simulink model "TerrainSimRunner"  (R2021a)
settings: Solver=VariableStepAuto  StartTime=0.0  StopTime=10.6  RelTol=1e-3
values from neighbouring files (symbols this model uses):
  init_parameters = struct    [TerrainGenerator.m]    (also in WorkspaceLoader.m = load('init_parameters'))
undefined symbols (not defined in the file or in its folder): Xref
libraries: vrlib x3
settings Model: Creator=16109  LastModifiedBy=16109

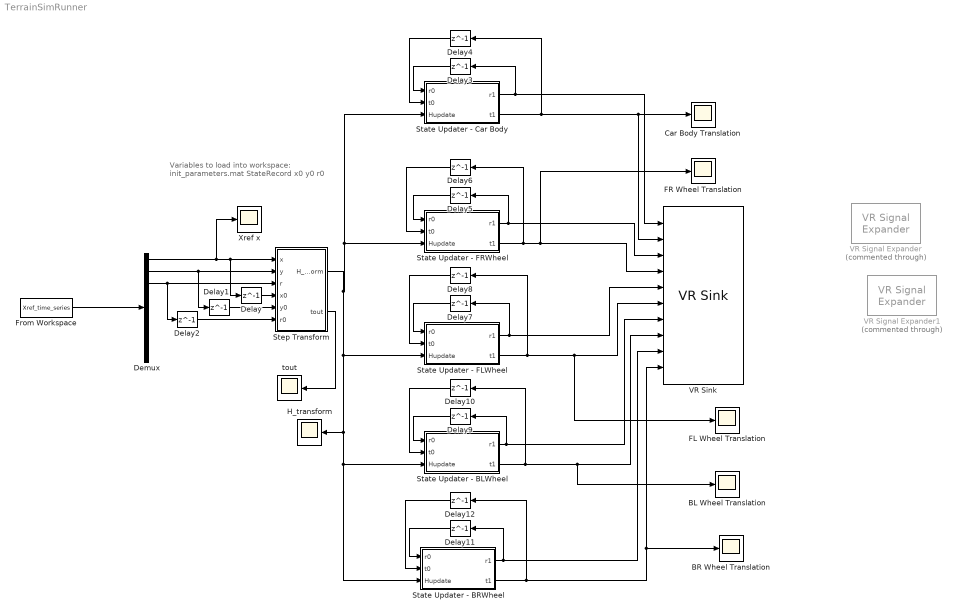
== system TerrainSimRunner ==
  note: Variables to load into workspace:
      | init_parameters.mat
      | StateRecord
      | x0
      | y0
      | r0
  BL Wheel Translation : Scope
  BR Wheel Translation : Scope
  Car Body Translation : Scope
  Delay : Delay  DelayLength=1  InitialCondition=Xref(1,1)
  Delay1 : Delay  DelayLength=1  InitialCondition=Xref(2,1)
  Delay10 : Delay  DelayLength=1  InitialCondition=init_parameters.BLWheelTranslation
  Delay11 : Delay  DelayLength=1  InitialCondition=init_parameters.BRWheelRotation
  Delay12 : Delay  DelayLength=1  InitialCondition=init_parameters.BLWheelTranslation
  Delay2 : Delay  DelayLength=1  InitialCondition=Xref(3,1)
  Delay3 : Delay  DelayLength=1  InitialCondition=init_parameters.BodyRotation
  Delay4 : Delay  DelayLength=1  InitialCondition=init_parameters.BodyTranslation
  Delay5 : Delay  DelayLength=1  InitialCondition=init_parameters.FRWheelRotation
  Delay6 : Delay  DelayLength=1  InitialCondition=init_parameters.FRWheelTranslation
  Delay7 : Delay  DelayLength=1  InitialCondition=init_parameters.FLWheelRotation
  Delay8 : Delay  DelayLength=1  InitialCondition=init_parameters.FLWheelTranslation
  Delay9 : Delay  DelayLength=1  InitialCondition=init_parameters.BLWheelRotation
  Demux : Demux  Outputs=9
  FL Wheel Translation : Scope
  FR Wheel Translation : Scope
  From Workspace : FromWorkspace  VariableName=Xref_time_series
  H_transform : Scope
  State Updater - BLWheel : MATLAB Function  TreatAsAtomicUnit=on
  State Updater - BRWheel : MATLAB Function  TreatAsAtomicUnit=on
  State Updater - Car Body : MATLAB Function  TreatAsAtomicUnit=on
  State Updater - FLWheel : MATLAB Function  TreatAsAtomicUnit=on
  State Updater - FRWheel : MATLAB Function  TreatAsAtomicUnit=on
  Step Transform : MATLAB Function  TreatAsAtomicUnit=on
  VR Signal Expander : vrlib/VR Signal Expander  Commented=through  outwidth=4  outidx=[2 4]
  VR Signal Expander1 : vrlib/VR Signal Expander  Commented=through  outwidth=3  outidx=[1]
  VR Sink : vrlib/VR Sink  InstantiateOnLoad=on  SampleTime=0.1  ViewEnable=on  RemoteChange=off  RemoteView=off  FieldsWritten=CarBody.rotation.4.1.1.double#CarBody.translation.3.1.1.double#FRWheel.rotation.4.1.1.double#FRWheel.translation.3.1.1.double#FLWheel.rotation.4.1.1.double#FLWheel.translation.3.1.1.double#BLWheel.rotation.4.1.1.double#BLWheel.translation.3.1.1.double#BRWheel.rotation.4.1.1.double#BRWheel.translation.3.1.1.double  WorldFileName=TerrainSimulation.x3d  AutoView=off  VideoDimensions=[]  AllowVariableSize=off  FigureProperties="{'Position', 'Name', 'Viewpoint', 'CameraBound', 'CameraDirection', 'CameraPosition', 'CameraUpVector', 'ZoomFactor', 'Antialiasing', 'Headlight', 'Lighting', 'NavPanel', 'Sound', 'StatusBar', 'Stereo3D', 'Stereo3DCameraOffset', 'Stereo3DHIT', 'ToolBar', 'Textures', 'Transparency', 'Triad', 'Wireframe', 'NavZones', 'NavMode', 'NavSpeed', 'CaptureFileFormat', 'CaptureFileName', 'Record2DCompressMethod', 'Record2DCompressQuality', 'Record2D', 'Record2DFileName', 'Record2DFPS'; [5.0000000000000000e+00   9.2000000000000000e+01   5.7600000000000000e+02   3.5000000000000000e+02], '', 'Terrain_Viewpoint_1', 'on', [-6.3529519425843139e-01   3.7869028019551818e-02  -7.7134036123425920e-01], [8.6325161926899163e+00  -2.3623592187623753e+01  -3.9838539482567555e+01], [-3.3509979340254042e-02   9.9650453597280886e-01   7.6523140750056506e-02], [1.0000000000000000e+00], 'off', 'on', 'on', 'halfbar', 'on', 'on', 'off', [1.0000000149011612e-01], [0.0000000000000000e+00], 'on', 'on', 'on', 'none', 'off', 'off', 'examine', 'normal', 'tif', '%f_anim_%n.tif', 'auto', [7.5000000000000000e+01], 'off', '%f_anim_%n.avi', 'auto'}"
  Xref x : Scope
  tout : Scope
  wires:
  From Workspace/1 -> Demux/1
  Demux/1 -> Xref x/1, Delay/1, Step Transform/1(x)
  Demux/2 -> Delay1/1, Step Transform/2(y)
  Demux/3 -> Delay2/1, Step Transform/3(r)
  Delay/1 -> Step Transform/4(x0)
  Delay1/1 -> Step Transform/5(y0)
  Delay2/1 -> Step Transform/6(r0)
  Step Transform/1(H_transform) -> H_transform/1, State Updater - BRWheel/3(Hupdate), State Updater - BLWheel/3(Hupdate), State Updater - FLWheel/3(Hupdate), State Updater - FRWheel/3(Hupdate), State Updater - Car Body/3(Hupdate)
  State Updater - Car Body/1(r1) -> Delay3/1, VR Sink/1
  State Updater - Car Body/2(t1) -> Delay4/1, VR Sink/2, Car Body Translation/1
  State Updater - FRWheel/1(r1) -> Delay5/1, VR Sink/3
  State Updater - FRWheel/2(t1) -> Delay6/1, FR Wheel Translation/1, VR Sink/4
  State Updater - FLWheel/1(r1) -> Delay7/1, VR Sink/5
  State Updater - FLWheel/2(t1) -> Delay8/1, FL Wheel Translation/1, VR Sink/6
  State Updater - BLWheel/1(r1) -> Delay9/1, VR Sink/7
  State Updater - BLWheel/2(t1) -> Delay10/1, BL Wheel Translation/1, VR Sink/8
  State Updater - BRWheel/1(r1) -> Delay11/1, VR Sink/9
  State Updater - BRWheel/2(t1) -> Delay12/1, BR Wheel Translation/1, VR Sink/10
  Delay3/1 -> State Updater - Car Body/1(r0)
  Delay4/1 -> State Updater - Car Body/2(t0)
  Delay5/1 -> State Updater - FRWheel/1(r0)
  Delay6/1 -> State Updater - FRWheel/2(t0)
  Delay7/1 -> State Updater - FLWheel/1(r0)
  Delay8/1 -> State Updater - FLWheel/2(t0)
  Delay9/1 -> State Updater - BLWheel/1(r0)
  Delay10/1 -> State Updater - BLWheel/2(t0)
  Delay11/1 -> State Updater - BRWheel/1(r0)
  Delay12/1 -> State Updater - BRWheel/2(t0)
  Step Transform/2(tout) -> tout/1

== matlab function TerrainSimRunner/State Updater - Car Body ==
  data: r0 input; t0 input; r1 output; Hupdate input; t1 output
function [r1, t1]= fcn(r0, t0,Hupdate)
Hupdate_reshaped = eye(4);
Hupdate_reshaped(1,:) = Hupdate(1:4);
Hupdate_reshaped(2,:) = Hupdate(5:8);
Hupdate_reshaped(3,:) = Hupdate(9:12);
H0 = eye(4);
H0(1:3,1:3) = axang2rotm(r0');
H0(1:3,4) = t0;
H1 = Hupdate_reshaped * H0;
r1 = rotm2axang(H1(1:3,1:3))';
t1 = H0(1:3,4);
end

== matlab function TerrainSimRunner/Step Transform ==
  data: x input; H_transform output; y input; r input; x0 input; y0 input; r0 input; tout output
function [H_transform, tout]= fcn(x, y, r, x0, y0, r0)
H_transform0 = eye(4);
H_transform0(1,:) = [cos(r-r0), -sin(r-r0), 0, x-x0];
H_transform0(2,:) = [sin(r-r0), cos(r-r0), 0, y-y0];
% H_transform = [
%     cos(r-r0), -sin(r-r0), 0, x-x0;
%     sin(r-r0), cos(r-r0), 0, y-y0;
%     0, 0, 1, 0;
%     0, 0, 0, 1];
H_transform = reshape(H_transform0,[1,16])';
tout = [x-x0, y-y0, 0];
end

== matlab function TerrainSimRunner/State Updater - FRWheel ==
  data: r0 input; t0 input; r1 output; Hupdate input; t1 output
function [r1, t1]= fcn(r0, t0,Hupdate)
Hupdate_reshaped = eye(4);
Hupdate_reshaped(1,:) = Hupdate(1:4);
Hupdate_reshaped(2,:) = Hupdate(5:8);
Hupdate_reshaped(3,:) = Hupdate(9:12);
H0 = eye(4);
H0(1:3,1:3) = axang2rotm(r0');
H0(1:3,4) = t0;
H1 = Hupdate_reshaped * H0;
r1 = rotm2axang(H1(1:3,1:3))';
t1 = H0(1:3,4);
end

== matlab function TerrainSimRunner/State Updater - FLWheel ==
  data: r0 input; t0 input; r1 output; Hupdate input; t1 output
function [r1, t1]= fcn(r0, t0,Hupdate)
Hupdate_reshaped = eye(4);
Hupdate_reshaped(1,:) = Hupdate(1:4);
Hupdate_reshaped(2,:) = Hupdate(5:8);
Hupdate_reshaped(3,:) = Hupdate(9:12);
H0 = eye(4);
H0(1:3,1:3) = axang2rotm(r0');
H0(1:3,4) = t0;
H1 = Hupdate_reshaped * H0;
r1 = rotm2axang(H1(1:3,1:3))';
t1 = H0(1:3,4);
end

== matlab function TerrainSimRunner/State Updater - BLWheel ==
  data: r0 input; t0 input; r1 output; Hupdate input; t1 output
function [r1, t1]= fcn(r0, t0,Hupdate)
Hupdate_reshaped = eye(4);
Hupdate_reshaped(1,:) = Hupdate(1:4);
Hupdate_reshaped(2,:) = Hupdate(5:8);
Hupdate_reshaped(3,:) = Hupdate(9:12);
H0 = eye(4);
H0(1:3,1:3) = axang2rotm(r0');
H0(1:3,4) = t0;
H1 = Hupdate_reshaped * H0;
r1 = rotm2axang(H1(1:3,1:3))';
t1 = H0(1:3,4);
end

== matlab function TerrainSimRunner/State Updater - BRWheel ==
  data: r0 input; t0 input; r1 output; Hupdate input; t1 output
function [r1, t1]= fcn(r0, t0,Hupdate)
Hupdate_reshaped = eye(4);
Hupdate_reshaped(1,:) = Hupdate(1:4);
Hupdate_reshaped(2,:) = Hupdate(5:8);
Hupdate_reshaped(3,:) = Hupdate(9:12);
H0 = eye(4);
H0(1:3,1:3) = axang2rotm(r0');
H0(1:3,4) = t0;
H1 = Hupdate_reshaped * H0;
r1 = rotm2axang(H1(1:3,1:3))';
t1 = H0(1:3,4);
end
